simulink library "WDB2Weather"  (Simulink 7.6)
settings: Solver=ode45  StartTime=0.0  StopTime=10.0  RelTol=1e-3
settings Model: Creator=lena.frank  LastModifiedBy=awohlfei

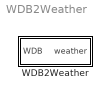
== system WDB2Weather ==
  WDB2Weather : Subsystem
      mask Type: WDB 2 weather
      mask Description:
      | Creates the weather data vector from the weather data bus WDB.
      | Format in weather data vector:
      | 1  timevalue (comment line) format YYYYMMDDHHMM    -
      | 2  zenith angle of sun (at time, not averaged)       degree
      | 3  azimuth angle of sun (0°=south, east negative) degree
      | 4  beam solar radiation on a normal surface         W/m^2
      | 5  diffuse solar radiation on a horizontal surface   W/m^2
      | 6  ambient temperature                                    degree celsius
      | 7  radiation temperature of sky                          degree celsius
      | 8  relative humidity                                           percent
      | 9  precipitation                                                 m/s
      | 10 cloud index (0=no cloud, 1=covered sky)         -
      | 11 station pressure                                           Pa
      | 12 mean wind speed                                         m/s
      | 13 wind direction (north=0° west=270°)             degree
      | 14 incidence angle on surface (0° = vertical)      degree
      | 15 longitudinal incidence angle                       degree
      | 16 transversal incidence angle                        degree
      | 17 direct solar radiation on surface                 W/m²
      | 18 diffuse solar radiation on surface                W/m²

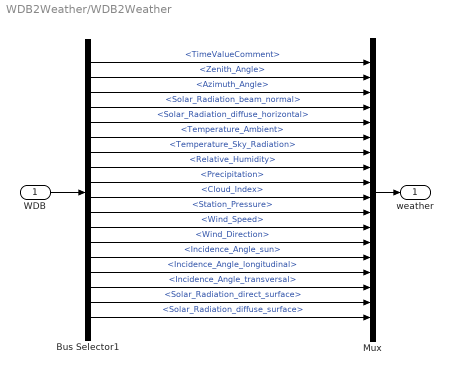
== system WDB2Weather/WDB2Weather ==
  WDB : Inport
  Bus Selector1 : BusSelector  OutputSignals=TimeValueComment,Zenith_Angle,Azimuth_Angle,Solar_Radiation_beam_normal,Solar_Radiation_diffuse_horizontal,Temperature_Ambient,Temperature_Sky_Radiation,Relative_Humidity,Precipitation,Cloud_Index,Station_Pressure,Wind_Speed,Wind_Direction,Incidence_Angle_sun,Incidence_Angle_longitudinal,Incidence_Angle_transversal,Solar_Radiation_direct_surface,Solar_Radiation_diffuse_surface
  Mux : Mux  Inputs=18
  weather : Outport
  wires:
  Mux/1 -> weather/1
  WDB/1 -> Bus Selector1/1
  Bus Selector1/18 -> Mux/18  "<Solar_Radiation_diffuse_surface>"
  Bus Selector1/17 -> Mux/17  "<Solar_Radiation_direct_surface>"
  Bus Selector1/16 -> Mux/16  "<Incidence_Angle_transversal>"
  Bus Selector1/15 -> Mux/15  "<Incidence_Angle_longitudinal>"
  Bus Selector1/14 -> Mux/14  "<Incidence_Angle_sun>"
  Bus Selector1/13 -> Mux/13  "<Wind_Direction>"
  Bus Selector1/12 -> Mux/12  "<Wind_Speed>"
  Bus Selector1/11 -> Mux/11  "<Station_Pressure>"
  Bus Selector1/10 -> Mux/10  "<Cloud_Index>"
  Bus Selector1/9 -> Mux/9  "<Precipitation>"
  Bus Selector1/8 -> Mux/8  "<Relative_Humidity>"
  Bus Selector1/7 -> Mux/7  "<Temperature_Sky_Radiation>"
  Bus Selector1/6 -> Mux/6  "<Temperature_Ambient>"
  Bus Selector1/5 -> Mux/5  "<Solar_Radiation_diffuse_horizontal>"
  Bus Selector1/4 -> Mux/4  "<Solar_Radiation_beam_normal>"
  Bus Selector1/3 -> Mux/3  "<Azimuth_Angle>"
  Bus Selector1/2 -> Mux/2  "<Zenith_Angle>"
  Bus Selector1/1 -> Mux/1  "<TimeValueComment>"
